simulink library "rw_motor_lib"  (R2018b)
settings: Solver=VariableStepAuto  StartTime=0.0  StopTime=10.0  RelTol=1e-3
undefined symbols (not defined in the file): simParams
libraries: simulink x1
settings Model: Creator=Taylor  LastModifiedBy=Taylor
settings SFSimCC: SimUseLocalCustomCode=off
settings RTWCC: RTWUseLocalCustomCode=off
settings CodeAppCC: StateflowObjectComments=on

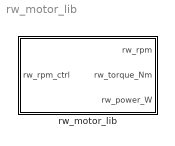
== system rw_motor_lib ==
  rw_motor_lib : Subsystem

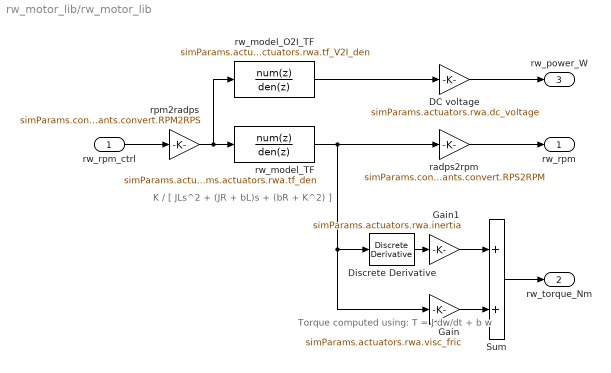
== system rw_motor_lib/rw_motor_lib ==
  note: K / [ JLs^2 + (JR + bL)s + (bR + K^2) ]
  note: Torque computed using: T = J dw/dt + b w
  rw_rpm_ctrl : Inport
  DC voltage : Gain  Gain=simParams.actuators.rwa.dc_voltage
  Discrete Derivative : simulink/Discrete/Discrete Derivative  gainval=1.0  ICPrevScaledInput=simParams.actuators.rwa.ic.deriv1  OutMin=[]  OutMax=[]  OutDataType=fixdt(1, 16)  OutScaling=2^-10  DoSatur=off
  Gain : Gain  Gain=simParams.actuators.rwa.visc_fric
  Gain1 : Gain  Gain=simParams.actuators.rwa.inertia
  Sum : Sum
  radps2rpm : Gain  Gain=simParams.constants.convert.RPS2RPM
  rpm2radps : Gain  Gain=simParams.constants.convert.RPM2RPS
  rw_model_O2I_TF : DiscreteTransferFcn  Numerator=simParams.actuators.rwa.tf_V2I_num  Denominator=simParams.actuators.rwa.tf_V2I_den
  rw_model_TF : DiscreteTransferFcn  Numerator=simParams.actuators.rwa.tf_num  Denominator=simParams.actuators.rwa.tf_den
  rw_rpm : Outport
  rw_torque_Nm : Outport  Port=2
  rw_power_W : Outport  Port=3
  wires:
  DC voltage/1 -> rw_power_W/1
  rw_model_O2I_TF/1 -> DC voltage/1
  radps2rpm/1 -> rw_rpm/1
  rpm2radps/1 -> rw_model_TF/1, rw_model_O2I_TF/1
  Sum/1 -> rw_torque_Nm/1
  Gain/1 -> Sum/2
  Gain1/1 -> Sum/1
  Discrete Derivative/1 -> Gain1/1
  rw_rpm_ctrl/1 -> rpm2radps/1
  rw_model_TF/1 -> radps2rpm/1, Discrete Derivative/1, Gain/1
